simulink model "SG8_MPC_simu_MPC_validation_2018"  (R2018b)
settings: Solver=ode45  SolverName=ode5  StartTime=0.0  StopTime=10  RelTol=1e-3  EnableMultiTasking=on
undefined symbols (not defined in the file): A_OBS, Amaxpred, Arefpred, B_OBS, Bmaxpred, Brefpred, C_OBS, Cmaxpred, Crefpred, D_OBS, Dmaxpred, Drefpred, F, H, lambda_e, lambda_u, National_Instruments, Np, PCIe, sigbuilder_block, sldrtexcb_modeswitch, Te
libraries: sldrtlib x2
Description:
  | Real-Time Controller
  | 
  | The example model "sldrtex_controller" shows how to build a simple closed-loop real-time controller using
  | Simulink Desktop Real-Time. The output of the controlled plant is connected
  | to the analog input of your data acquisition board. This signal is subtracted from
  | the set point value generated by the signal generator and processed by a PID
  | controller. The output of the controller drives the input of the plant using the analog
  | output of your data acquisition board.
  | 
  | This model is a simplified version of the controller used for the CE152 Magnetic
  | Levitation Model.
  | 
  | How to run this model in Normal Mode:
  | 
  | 1) Open the Analog Input and Analog Output blocks and select your data acquisition
  |    board. If there's no board installed, install it using the Install new board button.
  | 2) Double-click the orange button to switch to Normal Mode if needed.
  | 3) Start the real-time execution using Simulation->Run.
  | 
  | How to run this model in External Mode:
  | 
  | 1) Open the Analog Input and Analog Output blocks and select your data acquisition
  |    board. If there's no board installed, install it using the Install new board button.
  | 2) Double-click the orange button to switch to External Mode if needed.
  | 3) Start the real-time execution using Simulation->Run. The model will automatically
  |    build, connect to Simulink in External Mode and start.
  | 
  | Note:
  | To run this model, you must have a data acquisition board connected to your
  |    computer.
settings Model: SimulationMode=external  ExtModeTrigDuration=100000  Creator=The MathWorks, Inc.  LastModifiedBy=ouyang
settings SolverCC: AutoInsertRateTranBlk=on
settings DataIOCC: LimitDataPoints=on  SaveFormat=Array  SignalLoggingName=logsOut
settings OptimizationCC: ExpressionDepthLimit=2147483647  InitFltsAndDblsToZero=on  EfficientMapNaN2IntZero=off  LifeSpan=inf
settings DebuggingCC: UnderspecifiedInitializationDetection=Classic  MergeDetectMultiDrivingBlocksExec=none  SignalResolutionControl=TryResolveAllWithWarning  FcnCallInpInsideContextMsg=warning  AllowSymbolicDim=off  StateNameClashWarn=warning  SFUnexpectedBacktrackingDiag=warning  SFNoUnconditionalDefaultTransitionDiag=warning  SFExecutionAtInitializationDiag=none
settings HardwareCC: TargetBitPerLong=64  TargetBitPerPointer=64  TargetBitPerSizeT=64  TargetBitPerPtrDiffT=64  TargetIntDivRoundTo=Zero  TargetEndianess=LittleEndian  TargetWordSize=64  TargetHWDeviceType=Intel->x86-64
settings ModelReferenceCC: PropagateSignalLabelsOutOfModel=off
settings SFSimCC: SimUseLocalCustomCode=off
settings RTWCC: Description=Simulink Desktop Real-Time  SystemTargetFile=sldrt.tlc  TemplateMakefile=sldrt.tmf  RTWUseLocalCustomCode=off  RTWCompilerOptimization=on
settings CodeAppCC: MaxIdLength=95  StateflowObjectComments=on
settings TargetCC: TargetPreCompLibLocation=C:\Program Files\MATLAB\R2019b\toolbox\sldrt\lib\win64
settings ConfigComp: CovMetricSettings=dw  CovSaveCumulativeToWorkspaceVar=on  CovSaveSingleToWorkspaceVar=on  CovExternalEMLEnable=off  CovSFcnEnable=off

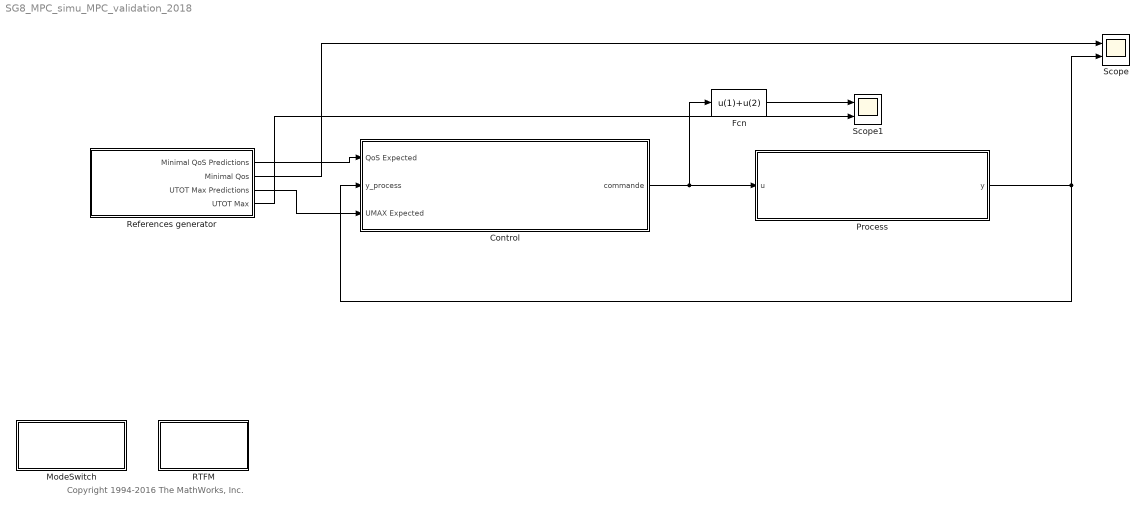
== system SG8_MPC_simu_MPC_validation_2018 ==
  note: Copyright 1994-2016 The MathWorks, Inc.
  Control : Subsystem
  Fcn : Fcn  Expr=u(1)+u(2)
  ModeSwitch : Subsystem  InitFcn=sldrtexcb_modeswitch('CheckKernel');  mask(Simulink Desktop Real-Time Example Mode Switch){}
      settings: OpenFcn=sldrtexcb_modeswitch(gcbh);
      mask Display: disp('Switch To\nNormal Mode');
  Process : Subsystem
  "RTFM " : Subsystem  mask(Simulink Desktop Real-Time Example Info){}
      settings: OpenFcn=web([docroot '/sldrt/examples/real-time-controller.html']);
      mask Display: disp('Info')
  References generator : Subsystem
  Scope : Scope  NumInputPorts=2
  Scope1 : Scope  NumInputPorts=2
  wires:
  Control/1(commande) -> Fcn/1, Process/1(u)
  References generator/1(Minimal QoS Predictions) -> Control/1(QoS Expected)
  References generator/2(Minimal Qos) -> Scope/1
  Fcn/1 -> Scope1/1
  Process/1(y) -> Scope/2, Control/2(y_process)
  References generator/4(UTOT Max) -> Scope1/2
  References generator/3(UTOT Max Predictions) -> Control/3(UMAX Expected)

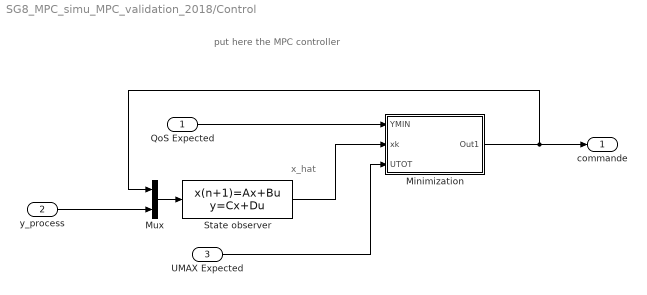
== system SG8_MPC_simu_MPC_validation_2018/Control ==
  note: x_hat
  note: put here the MPC controller
  QoS Expected : Inport
  y_process : Inport  Port=2
  UMAX Expected : Inport  Port=3
  Minimization : Subsystem
  Mux : Mux  Inputs=2
  State observer : DiscreteStateSpace  A=A_OBS  B=B_OBS  C=C_OBS  D=D_OBS  SampleTime=Te
  commande : Outport
  wires:
  y_process/1 -> Mux/2
  Mux/1 -> State observer/1
  Minimization/1(Out1) -> commande/1, Mux/1
  QoS Expected/1 -> Minimization/1(YMIN)
  State observer/1 -> Minimization/2(xk)
  UMAX Expected/1 -> Minimization/3(UTOT)

== system SG8_MPC_simu_MPC_validation_2018/ModeSwitch ==

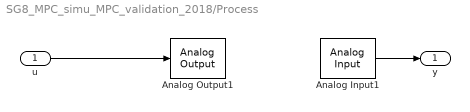
== system SG8_MPC_simu_MPC_validation_2018/Process ==
  u : Inport
  Analog Input1 : sldrtlib/Analog Input  SampleTime=Te  MaxMissedTicks=10  ShowMissedTicks=off  YieldWhenWaiting=off  DrvName=National_Instruments/PCIe-6323  DrvAddress=4294967295  DrvOptions=[0 0 0 0 0 0 0]  Channels=[1 2]  RangeMode=1  VoltRange=1  DataType=1
      settings: AttributesFormatString=National Instruments\nPCIe-6323 [auto]
  Analog Output1 : sldrtlib/Analog Output  SampleTime=Te  MaxMissedTicks=10  ShowMissedTicks=off  YieldWhenWaiting=off  DrvName=National_Instruments/PCIe-6323  DrvAddress=4294967295  DrvOptions=[0 0 0 0 0 0 0]  Channels=[1 2]  RangeMode=1  VoltRange=1  InitialValue=0  FinalValue=0
      settings: AttributesFormatString=National Instruments\nPCIe-6323 [auto]
  y : Outport
  wires:
  Analog Input1/1 -> y/1
  u/1 -> Analog Output1/1

== system SG8_MPC_simu_MPC_validation_2018/RTFM  ==

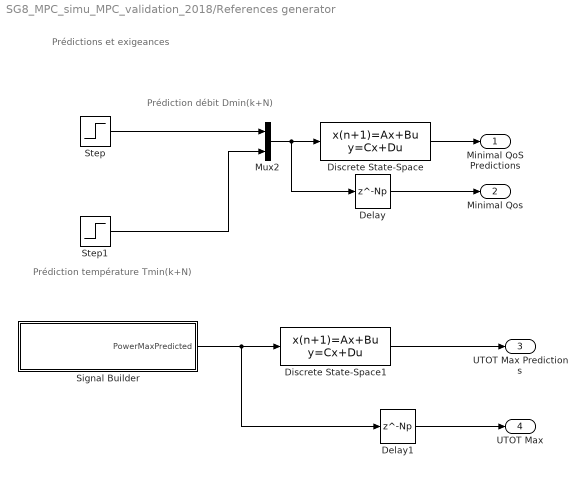
== system SG8_MPC_simu_MPC_validation_2018/References generator ==
  note: Prédiction débit Dmin(k+N)
  note: Prédictions et exigeances
  note: Prédiction température Tmin(k+N)
  Delay : Delay  DelayLength=Np  SampleTime=Te
  Delay1 : Delay  DelayLength=Np  InitialCondition=15  SampleTime=Te
  Discrete State-Space : DiscreteStateSpace  A=Arefpred  B=Brefpred  C=Crefpred  D=Drefpred  SampleTime=Te
  Discrete State-Space1 : DiscreteStateSpace  A=Amaxpred  B=Bmaxpred  C=Cmaxpred  D=Dmaxpred  InitialCondition=15*ones(Np,1)  SampleTime=Te
  Mux2 : Mux  Inputs=2
  Signal Builder : Subsystem  Tag=STV Subsys  LoadFcn=sigbuilder_block('load');  StartFcn=sigbuilder_block('start');  StopFcn=sigbuilder_block('stop');  ClipboardFcn=sigbuilder_block('clipboard');  mask(Sigbuilder block){tuvar=[0:10]}
      mask help: Simulink:masks:SigbuilderBlock_MD
      mask init:
      | if ~strcmp(get_param(bdroot(gcbh),'SimulationStatus'),'stopped') tuvar = sigbuilder_block('maskInit'); end
      settings: CopyFcn=sigbuilder_block('copy');  DeleteFcn=sigbuilder_block('delete');  ModelCloseFcn=sigbuilder_block('modelClose');  PreSaveFcn=sigbuilder_block('preSave');  PauseFcn=sigbuilder_block('pause');  ContinueFcn=sigbuilder_block('continue');  NameChangeFcn=sigbuilder_block('namechange');  OpenFcn=sigbuilder_block('open',[147.75 264 550.5 359.25 ]);  CloseFcn=sigbuilder_block('close');
      mask Display: plot(0, 0, 100, 100,[2, 2, 32, 32, 2], [68, 8, 8, 68, 68],[32, 2], [38, 38], [32, 19, 2],[53, 60, 44], [32, 17, 17, 2],[16, 16, 31, 31]);txt = getActiveGroup(gcbh);text(2, 100, txt,'verticalAlignment', 'top');
  Step : Step  Time=3  Before=5  After=5.5  SampleTime=0
  Step1 : Step  Time=7  Before=3  After=3  SampleTime=0
  Minimal QoS Predictions : Outport
  Minimal Qos : Outport  Port=2
  UTOT Max Predictions : Outport  Port=3
  UTOT Max : Outport  Port=4
  wires:
  Step/1 -> Mux2/1
  Step1/1 -> Mux2/2
  Mux2/1 -> Delay/1, Discrete State-Space/1
  Discrete State-Space/1 -> Minimal QoS Predictions/1
  Delay/1 -> Minimal Qos/1
  Signal Builder/1(PowerMaxPredicted) -> Delay1/1, Discrete State-Space1/1
  Discrete State-Space1/1 -> UTOT Max Predictions/1
  Delay1/1 -> UTOT Max/1

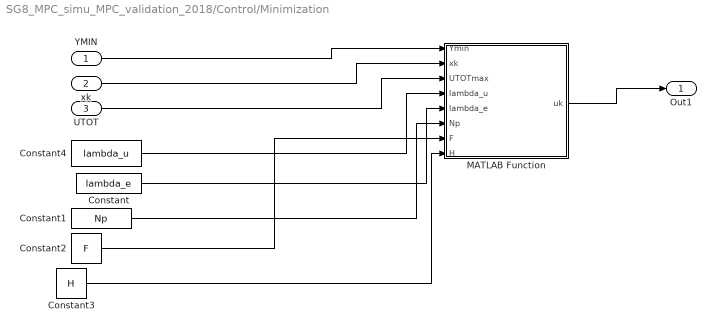
== system SG8_MPC_simu_MPC_validation_2018/Control/Minimization ==
  YMIN : Inport
  xk : Inport  Port=2
  UTOT : Inport  Port=3
  Constant : Constant  Value=lambda_e
  Constant1 : Constant  Value=Np
  Constant2 : Constant  Value=F
  Constant3 : Constant  Value=H
  Constant4 : Constant  Value=lambda_u  VectorParams1D=off
  MATLAB Function : MATLAB Function  TreatAsAtomicUnit=on
  Out1 : Outport
  wires:
  xk/1 -> MATLAB Function/2(xk)
  YMIN/1 -> MATLAB Function/1(Ymin)
  MATLAB Function/1(uk) -> Out1/1
  UTOT/1 -> MATLAB Function/3(UTOTmax)
  Constant4/1 -> MATLAB Function/4(lambda_u)
  Constant/1 -> MATLAB Function/5(lambda_e)
  Constant1/1 -> MATLAB Function/6(Np)
  Constant2/1 -> MATLAB Function/7(F)
  Constant3/1 -> MATLAB Function/8(H)

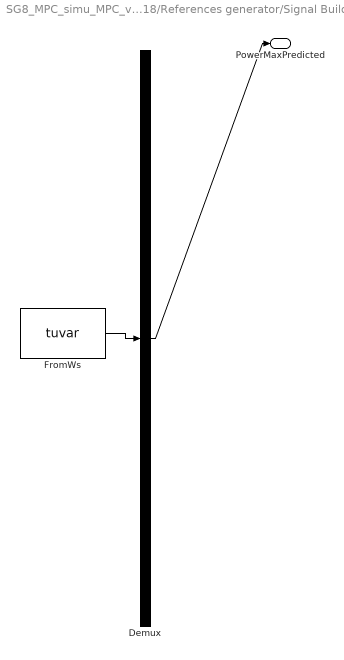
== system SG8_MPC_simu_MPC_validation_2018/References generator/Signal Builder ==
  Demux : Demux  Tag=STV Demux  Outputs=1
      settings: DisplayOption=none
  FromWs : FromWorkspace  Tag=STV FromWs  VariableName=tuvar
      SigBuilderData=|
      | common.afterFinalStr = 'Extrapolate'
      | common.sampleTime = 0
      | dataSet.timeRange = [0 20]
      | dataSet.name = 'Group 1'
      | sbobj.Groups.Name = 'Group 1'
      | sbobj.Groups.Signals.Name = 'PowerMaxPredicted'
      | sbobj.Groups.Signals.XData = [0 4 4 5.5 5.5 9 9 10.5 10.5 15 15 16 16 20]
      | sbobj.Groups.Signals.YData = [15 15 8 8 15 15 8 8 15 15 10 10 15 15]
      | sbobj.Groups.TimeRange = [0 20]
  PowerMaxPredicted : Outport  Tag=STV Outport
  wires:
  FromWs/1 -> Demux/1
  Demux/1 -> PowerMaxPredicted/1

== matlab function SG8_MPC_simu_MPC_validation_2018/Control/Minimization/MATLAB Function ==
  data: Ymin input; uk output; xk input; UTOTmax input; lambda_u input; lambda_e input; Np input; F input; H input
function uk = fcn(Ymin,xk,UTOTmax,lambda_u,lambda_e, Np, F,H)

uk = [0;0];
coder.extrinsic('quadprog');

% define H and f in quadprog
W = [eye(2*Np), zeros(2*Np,5*Np); zeros(2*Np), lambda_u*eye(2*Np), zeros(2*Np,3*Np); zeros(3*Np,4*Np), lambda_e*eye(3*Np)];
f = [-Ymin', zeros(1,5*Np)];

% define A in quadprog
T = zeros(Np,2*Np);
for i = 1:Np
    T(i,2*i-1:2*i) = [1,1];
end

P = zeros(Np,2*Np);
for i = 1:Np
    P(i,2*i) = 1;
end

Q = zeros(2*Np,3*Np);
for i = 1:Np
    Q(2*i-1,3*i-2) = 1;
    Q(2*i,3*i-1) = 1;
end

R = zeros(Np,3*Np);
for i = 1:Np
    R(i,3*i) = 1;
end

% lb = zeros(7*Np,1);
% ub = zeros(7*Np,1);
% lb(2*Np+1:4*Np,1) = -10;
% ub(2*Np+1:4*Np,1) = 10;
lb = [];
ub = [];

A = [zeros(Np,2*Np), T, zeros(Np,3*Np); -eye(2*Np), zeros(2*Np), -Q; P, zeros(Np,2*Np), -R];
b = [UTOTmax; -Ymin; P*Ymin + 2*ones(Np,1)];

% Aeq and beq in quadprog 
Aeq = [eye(2*Np), -H, zeros(2*Np,3*Np)];
beq = F*xk;

[Uopt] = quadprog(W,f,A,b,Aeq,beq,lb,ub);

uk = Uopt(2*Np+1:2*Np+2,1)
uk_tot = uk(1)+uk(2)
